simulink model "untitled1"  (R2022a)
settings: Solver=ode4  StartTime=0.0  StopTime=50000  FixedStep=1  RelTol=1e-3
libraries: nesl_utility x13, sm_lib x11, sharedtransform x4, sharedutil x1
settings Model: Creator=sakur  LastModifiedBy=sakur

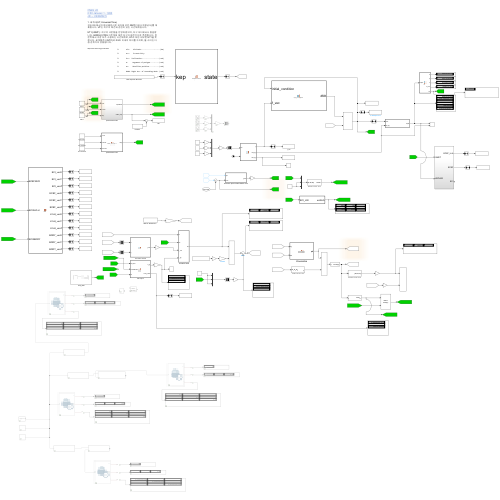
[thumbnail: Simulink's stored preview of the top-level diagram]
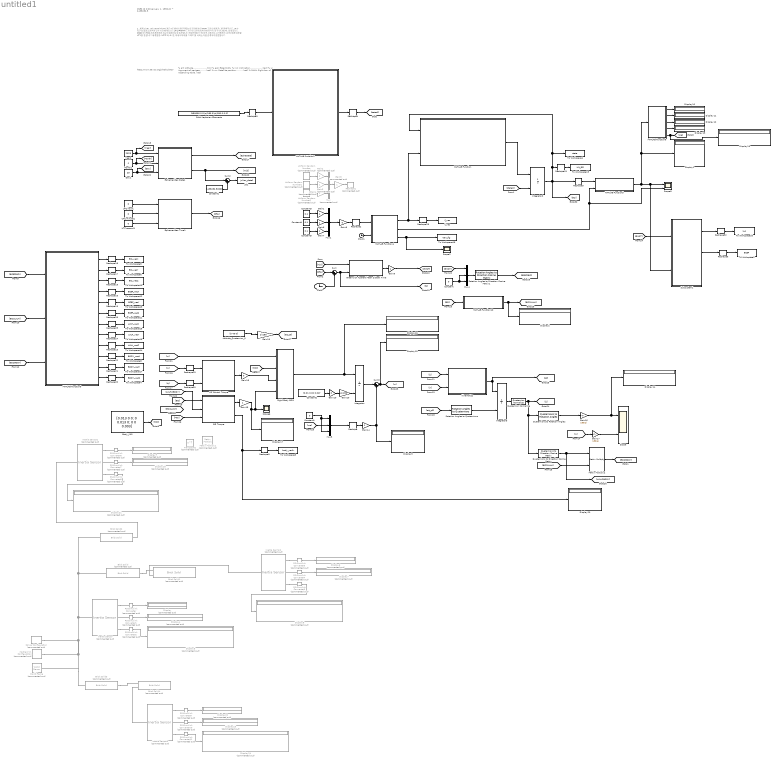
== system untitled1 ==
  note: % alt: Altitude.....................(Km)
      | % ecc: Eccentricity
      | % inc: Inclination...................(rad)
      | % w: Argument of perigee..........(rad)
      | % nu: Satellite position...........(rad) % RAAN: Right Asc. of Ascending Node. (rad)
  note: 1. 세계시(UT, Universal Time)
      | 경도 0도에서의 평균태양시로 과거에 쓰던 GMT(그리니치평균시)를 대체합니다. UT는 지구의 회전과 관련이 있는 시간체계입니다.
      |
      | UT1(=GMT) : 지구의 극운동을 반영하였으며, 지구 어디에서나 동일합니다. GCRS와 ITRS 기준계에 대한 지구의 회전각으로 측정합니다. 천문학에서 가장 자주 사용하는 시간체계로, UT라 하면 대부분 UT1을 뜻합니다. 세계협정시(UTC)와 0.9초 이내의 차이를 가지며, 둘 사이는 다음 관계식이 성립됩니다.
  note: CNES JD
      | 0:00 January 1, 1950
      | JD − 2433282.5
  note: https://www.aavso.org/jd-calculator
  Attitude_Quaternion_0 : Constant  Value=[0 45 0]'
  Body_MOI : Constant  Value=[0.013 0 0; 0 0.013 0; 0 0 0.003]
  Brick Solid : sm_lib/Body Elements/Brick Solid  Commented=on  GraphicAmbientColor=[0.15 0.15 0.15 1.0]  BasedOnType=Mass  BrickDimensions=[10 10 10]  BrickDimensionUnits=cm  CenterOfMass=[0 0 0]  CenterOfMassUnits=m  GraphicDiffuseColor=[0.5 0.5 0.5]  Density=1000  DensityUnits=kg/m^3  DoExposeReferenceFrame=on  GraphicEmissiveColor=[0.0 0.0 0.0 1.0]  ExportEntireGeometry=off  SerializedFrames=<Frames><Frame><Id>Frame1</Id><Value><Name>MS_Mount_F</Name><Origin><Source>GeometricFeature</Source><FeatureName>+z surface</FeatureName></Origin><PrimaryAxis><DefinedDirection>+Z</DefinedDirection><Source>ReferenceFrame</Source><SourceDirection>+Z</SourceDirection><FeatureName></FeatureName></PrimaryAxis><SecondaryAxis><DefinedDirection>+X</DefinedDirection><Source>ReferenceFrame</Source><SourceDirection>+X</SourceDirection><FeatureName></FeatureName></SecondaryAxis></Value></Frame></Frames>  MarkerShape=Sphere  MarkerSize=10  GraphicType=FromGeometry  InertiaType=CalculateFromGeometry  Mass=10  MassUnits=kg  MomentsOfInertia=[1 1 1]  MomentsOfInertiaUnits=kg*m^2  GraphicOpacity=1.0  ProductsOfInertia=[0 0 0]  ProductsOfInertiaUnits=kg*m^2  GraphicShininess=75  GraphicSpecularColor=[0.5 0.5 0.5 1.0]  GraphicVisPropType=SimpleVisualProperties
  Brick Solid1 : sm_lib/Body Elements/Brick Solid  Commented=on  GraphicAmbientColor=[0.15 0.15 0.15 1.0]  BasedOnType=Mass  BrickDimensions=[10 10 20]  BrickDimensionUnits=cm  CenterOfMass=[0 0 0]  CenterOfMassUnits=m  GraphicDiffuseColor=[0.5 0.5 0.5]  Density=1000  DensityUnits=kg/m^3  DoExposeReferenceFrame=on  GraphicEmissiveColor=[0.0 0.0 0.0 1.0]  ExportEntireGeometry=off  SerializedFrames=<Frames><Frame><Id>Frame1</Id><Value><Name>Mount_F</Name><Origin><Source>GeometricFeature</Source><FeatureName>-z surface</FeatureName></Origin><PrimaryAxis><DefinedDirection>+Z</DefinedDirection><Source>ReferenceFrame</Source><SourceDirection>+Z</SourceDirection><FeatureName></FeatureName></PrimaryAxis><SecondaryAxis><DefinedDirection>+X</DefinedDirection><Source>ReferenceFrame</Source><SourceDirection>+X</SourceDirection><FeatureName></FeatureName></SecondaryAxis></Value></Frame><Frame><Id>Frame2</Id><Value><Name>MOI_F</Name><Origin><Source>CenterOfMassFrame</Source><FeatureName></FeatureName></Origin><PrimaryAxis><DefinedDirection>-Z</DefinedDirection><Source>ReferenceFrame</Source><SourceDirection>+Z</SourceDirection><FeatureName></FeatureName></PrimaryAxis><SecondaryAxis><DefinedDirection>+X</DefinedDirection><Source>ReferenceFrame</Source><SourceDirection>+X</SourceDirection><FeatureName></FeatureName></SecondaryAxis></Value></Frame></Frames>  MarkerShape=Sphere  MarkerSize=10  GraphicType=FromGeometry  InertiaType=CalculateFromGeometry  Mass=2  MassUnits=kg  MomentsOfInertia=[1 1 1]  MomentsOfInertiaUnits=kg*m^2  GraphicOpacity=1.0  ProductsOfInertia=[0 0 0]  ProductsOfInertiaUnits=kg*m^2  GraphicShininess=75  GraphicSpecularColor=[0.5 0.5 0.5 1.0]  GraphicVisPropType=SimpleVisualProperties
  Brick Solid2 : sm_lib/Body Elements/Brick Solid  Commented=on  GraphicAmbientColor=[0.15 0.15 0.15 1.0]  BasedOnType=Mass  BrickDimensions=[10 10 30]  BrickDimensionUnits=cm  CenterOfMass=[0 0 0]  CenterOfMassUnits=m  GraphicDiffuseColor=[0.5 0.5 0.5]  Density=1000  DensityUnits=kg/m^3  DoExposeReferenceFrame=on  GraphicEmissiveColor=[0.0 0.0 0.0 1.0]  ExportEntireGeometry=off  SerializedFrames=<Frames><Frame><Id>Frame1</Id><Value><Name>MS_Mount_F</Name><Origin><Source>GeometricFeature</Source><FeatureName>+z surface</FeatureName></Origin><PrimaryAxis><DefinedDirection>+Z</DefinedDirection><Source>ReferenceFrame</Source><SourceDirection>+Z</SourceDirection><FeatureName></FeatureName></PrimaryAxis><SecondaryAxis><DefinedDirection>+X</DefinedDirection><Source>ReferenceFrame</Source><SourceDirection>+X</SourceDirection><FeatureName></FeatureName></SecondaryAxis></Value></Frame></Frames>  MarkerShape=Sphere  MarkerSize=10  GraphicType=FromGeometry  InertiaType=CalculateFromGeometry  Mass=12  MassUnits=kg  MomentsOfInertia=[1 1 1]  MomentsOfInertiaUnits=kg*m^2  GraphicOpacity=1.0  ProductsOfInertia=[0 0 0]  ProductsOfInertiaUnits=kg*m^2  GraphicShininess=75  GraphicSpecularColor=[0.5 0.5 0.5 1.0]  GraphicVisPropType=SimpleVisualProperties
  Brick Solid3 : sm_lib/Body Elements/Brick Solid  Commented=on  GraphicAmbientColor=[0.15 0.15 0.15 1.0]  BasedOnType=Mass  BrickDimensions=[10 10 10]  BrickDimensionUnits=cm  CenterOfMass=[0 0 0]  CenterOfMassUnits=m  GraphicDiffuseColor=[0.5 0.5 0.5]  Density=1000  DensityUnits=kg/m^3  DoExposeReferenceFrame=on  GraphicEmissiveColor=[0.0 0.0 0.0 1.0]  ExportEntireGeometry=off  SerializedFrames=<Frames><Frame><Id>Frame1</Id><Value><Name>MS_Mount_F</Name><Origin><Source>GeometricFeature</Source><FeatureName>+z surface</FeatureName></Origin><PrimaryAxis><DefinedDirection>+Z</DefinedDirection><Source>ReferenceFrame</Source><SourceDirection>+Z</SourceDirection><FeatureName></FeatureName></PrimaryAxis><SecondaryAxis><DefinedDirection>+X</DefinedDirection><Source>ReferenceFrame</Source><SourceDirection>+X</SourceDirection><FeatureName></FeatureName></SecondaryAxis></Value></Frame></Frames>  MarkerShape=Sphere  MarkerSize=10  GraphicType=FromGeometry  InertiaType=CalculateFromGeometry  Mass=10  MassUnits=kg  MomentsOfInertia=[1 1 1]  MomentsOfInertiaUnits=kg*m^2  GraphicOpacity=1.0  ProductsOfInertia=[0 0 0]  ProductsOfInertiaUnits=kg*m^2  GraphicShininess=75  GraphicSpecularColor=[0.5 0.5 0.5 1.0]  GraphicVisPropType=SimpleVisualProperties
  Brick Solid4 : sm_lib/Body Elements/Brick Solid  Commented=on  GraphicAmbientColor=[0.15 0.15 0.15 1.0]  BasedOnType=Mass  BrickDimensions=[10 10 10]  BrickDimensionUnits=cm  CenterOfMass=[0 0 0]  CenterOfMassUnits=m  GraphicDiffuseColor=[0.5 0.5 0.5]  Density=1000  DensityUnits=kg/m^3  DoExposeReferenceFrame=on  GraphicEmissiveColor=[0.0 0.0 0.0 1.0]  ExportEntireGeometry=off  SerializedFrames=<Frames><Frame><Id>Frame1</Id><Value><Name>MS_Mount_F</Name><Origin><Source>GeometricFeature</Source><FeatureName>-z surface</FeatureName></Origin><PrimaryAxis><DefinedDirection>+Z</DefinedDirection><Source>ReferenceFrame</Source><SourceDirection>+Z</SourceDirection><FeatureName></FeatureName></PrimaryAxis><SecondaryAxis><DefinedDirection>+X</DefinedDirection><Source>ReferenceFrame</Source><SourceDirection>+X</SourceDirection><FeatureName></FeatureName></SecondaryAxis></Value></Frame><Frame><Id>Frame2</Id><Value><Name>MoI_F</Name><Origin><Source>CenterOfMassFrame</Source><FeatureName></FeatureName></Origin><PrimaryAxis><DefinedDirection>-Z</DefinedDirection><Source>ReferenceFrame</Source><SourceDirection>+Z</SourceDirection><FeatureName></FeatureName></PrimaryAxis><SecondaryAxis><DefinedDirection>+X</DefinedDirection><Source>ReferenceFrame</Source><SourceDirection>+X</SourceDirection><FeatureName></FeatureName></SecondaryAxis></Value></Frame></Frames>  MarkerShape=Sphere  MarkerSize=10  GraphicType=FromGeometry  InertiaType=CalculateFromGeometry  Mass=10  MassUnits=kg  MomentsOfInertia=[1 1 1]  MomentsOfInertiaUnits=kg*m^2  GraphicOpacity=1.0  ProductsOfInertia=[0 0 0]  ProductsOfInertiaUnits=kg*m^2  GraphicShininess=75  GraphicSpecularColor=[0.5 0.5 0.5 1.0]  GraphicVisPropType=SimpleVisualProperties
  Clock : Clock
  Clock1 : Clock
  Constant : Constant  Value=0
  Constant1 : Constant  Value=0
  Constant2 : Constant  Value=[0.01 0.02 0.01]'
  Constant3 : Constant  Value=0.1
  Constant4 : Constant  Value=0.1
  Constant5 : Constant  Value=0.1
  Day1 : Constant  Value=25
  Display{,4..9,18,21..24} (12 alike) : Display  Commented=on
  Display{1..3,10..17,19..20} (13 alike) : Display
  Ephemerides Date1 : Subsystem
  Ephemerides Time1 : MATLAB Function  TreatAsAtomicUnit=on
  GG Torque : MATLAB Function  TreatAsAtomicUnit=on
  Gain{1,6..7,9,14..15} (6 alike) : Gain
  Gain10 : Gain  Gain=0
  Gain16 : Gain  Gain=180/pi
  Gain17 : Gain  Gain=180/pi
  Gain18 : Gain  Gain=0
  Gain19 : Gain  Gain=pi/180
  Gain{2..5} (4 alike) : Gain  Commented=on
  Gain20 : Gain  Gain=pi/180
  Gain8 : Gain  Gain=0
  Greenwich Aparent Mean Sideral Time : MATLAB Function  TreatAsAtomicUnit=on
  Inertia Sensor : sm_lib/Body Elements/Inertia Sensor  Commented=on  SensorExtent=Mechanism  SpanWeldJoints=off  ExcludeGroundedBodies=off  MeasurementFrame=World  SenseMass=on  SenseCenterOfMass=on  SenseInertiaMatrix=on  SenseCenteredInertiaMatrix=off  SensePrincipalInertiaMatrix=off  SenseRotationMatrix=off  GraphicType=PrincipalInertiaFrame  PrincipalInertiaFrameSize=20  GraphicVisPropType=SimpleVisualProperties  GraphicDiffuseColor=[0.5 0.5 0.5]  GraphicSpecularColor=[0.5 0.5 0.5 1.0]  GraphicAmbientColor=[0.15 0.15 0.15 1.0]  GraphicEmissiveColor=[0.0 0.0 0.0 1.0]  GraphicShininess=75  GraphicOpacity=1.0
      settings: SourceProductBaseCode=MS
  Inertia Sensor1 : sm_lib/Body Elements/Inertia Sensor  Commented=on  SensorExtent=Mechanism  SpanWeldJoints=off  ExcludeGroundedBodies=off  MeasurementFrame=Attached  SenseMass=on  SenseCenterOfMass=on  SenseInertiaMatrix=on  SenseCenteredInertiaMatrix=off  SensePrincipalInertiaMatrix=off  SenseRotationMatrix=off  GraphicType=PrincipalInertiaFrame  PrincipalInertiaFrameSize=20  GraphicVisPropType=SimpleVisualProperties  GraphicDiffuseColor=[0.5 0.5 0.5]  GraphicSpecularColor=[0.5 0.5 0.5 1.0]  GraphicAmbientColor=[0.15 0.15 0.15 1.0]  GraphicEmissiveColor=[0.0 0.0 0.0 1.0]  GraphicShininess=75  GraphicOpacity=1.0
      settings: SourceProductBaseCode=MS
  Inertia Sensor2 : sm_lib/Body Elements/Inertia Sensor  Commented=on  SensorExtent=Mechanism  SpanWeldJoints=off  ExcludeGroundedBodies=off  MeasurementFrame=World  SenseMass=on  SenseCenterOfMass=on  SenseInertiaMatrix=on  SenseCenteredInertiaMatrix=off  SensePrincipalInertiaMatrix=off  SenseRotationMatrix=off  GraphicType=PrincipalInertiaFrame  PrincipalInertiaFrameSize=20  GraphicVisPropType=SimpleVisualProperties  GraphicDiffuseColor=[0.5 0.5 0.5]  GraphicSpecularColor=[0.5 0.5 0.5 1.0]  GraphicAmbientColor=[0.15 0.15 0.15 1.0]  GraphicEmissiveColor=[0.0 0.0 0.0 1.0]  GraphicShininess=75  GraphicOpacity=1.0
      settings: SourceProductBaseCode=MS
  Inertia Sensor3 : sm_lib/Body Elements/Inertia Sensor  Commented=on  SensorExtent=Mechanism  SpanWeldJoints=off  ExcludeGroundedBodies=off  MeasurementFrame=Attached  SenseMass=on  SenseCenterOfMass=on  SenseInertiaMatrix=on  SenseCenteredInertiaMatrix=off  SensePrincipalInertiaMatrix=off  SenseRotationMatrix=off  GraphicType=PrincipalInertiaFrame  PrincipalInertiaFrameSize=20  GraphicVisPropType=SimpleVisualProperties  GraphicDiffuseColor=[0.5 0.5 0.5]  GraphicSpecularColor=[0.5 0.5 0.5 1.0]  GraphicAmbientColor=[0.15 0.15 0.15 1.0]  GraphicEmissiveColor=[0.0 0.0 0.0 1.0]  GraphicShininess=75  GraphicOpacity=1.0
      settings: SourceProductBaseCode=MS
  Integrator : Integrator  InitialConditionSource=external
  Integrator2 : Integrator  InitialConditionSource=external  InitialCondition=[-7000 0 0 0 -9.175045 0 5233.5]'
  Integrator3 : Integrator  InitialConditionSource=external
  JD1 : ToWorkspace  VariableName=Julian_date1  SampleTime=-1
  Kinematics : MATLAB Function  TreatAsAtomicUnit=on
  MATLAB Function : MATLAB Function  TreatAsAtomicUnit=on
  MATLAB Function10 : MATLAB Function  TreatAsAtomicUnit=on
  MATLAB Function2 : MATLAB Function  TreatAsAtomicUnit=on
  MATLAB Function4 : MATLAB Function  TreatAsAtomicUnit=on
  MATLAB Function5 : MATLAB Function  TreatAsAtomicUnit=on
  MATLAB Function8 : MATLAB Function  TreatAsAtomicUnit=on
  MATLAB Function9 : MATLAB Function  TreatAsAtomicUnit=on
  Matrix Multiply1 : Product  Commented=on  Multiplication=Matrix(*)
  Matrix Multiply2 : Product  Multiplication=Matrix(*)
  Mechanism Configuration : sm_lib/Utilities/Mechanism Configuration  Commented=on  UniformGravity=None  GravityVector=[0 0 -9.80665]  GravityUnits=m/s^2  LinearizationDelta=0.001  JointModeTransitionNonlinearIterations=2
  Month1 : Constant  Value=4
  Mux : Mux  Commented=on  Inputs=3
  Mux1 : Mux  Inputs=3
  Mux4 : Mux  Inputs=3
  Mux5 : Mux  Inputs=3
  Orbit Keplerian Elements : Constant  Value=[450000 0 0*pi/180 0*pi/180 0 0 0]
  PD Control Torque : MATLAB Function  TreatAsAtomicUnit=on
  PS-Simulink Converter{,1..11} (12 alike) : nesl_utility/PS-Simulink Converter  Commented=on  PhysicalDomain=network_engine_domain  SubClassName=ps_output  LeftPortType=input  RightPortType=output  PseudoPeriodic=off  Frequencies=[]  VectorFormat=inherit  Unit=inherit  AffineConversion=off
      settings: SourceProductBaseCode=SS,PW,VE
  Quaternion Normalize : sharedutil/Quaternion Normalize  aMode=aMode
      settings: SourceProductBaseCode=AE,PW,DR,MT,VE
  Quaternions to Direction Cosine Matrix : sharedtransform/Quaternions to  Direction Cosine Matrix  aMode=aMode
      settings: SourceProductBaseCode=AE,PW,DR,MT,VE
  Quaternions to Rotation Angles : sharedtransform/Quaternions to Rotation Angles  rotationOrder=ZYX  aMode=aMode
      settings: SourceProductBaseCode=AE,PW,DR,MT,VE
  Reshape{,2,29..30} (4 alike) : Reshape  OutputDimensionality=Column vector (2-D)
  Reshape1 : Reshape  Commented=on  OutputDimensionality=Column vector (2-D)
  Reshape{3..6,9,13,16..26,28,31..32} (20 alike) : Reshape  OutputDimensionality=Row vector (2-D)
  Rigid Body EOM : MATLAB Function  TreatAsAtomicUnit=on
  Rotation Angles to Direction Cosine Matrix1 : sharedtransform/Rotation Angles to Direction Cosine Matrix  rotationOrder=ZYX  aMode=aMode
      settings: SourceProductBaseCode=AE,PW,DR,MT,VE
  Rotation Angles to Quaternions : sharedtransform/Rotation Angles to Quaternions  rotationOrder=ZYX  aMode=aMode
      settings: SourceProductBaseCode=AE,PW,DR,MT,VE
  Scope : Scope  NumInputPorts=2
  Scope2 : Scope
  Scope5 : Scope  NumInputPorts=2
  Scope6 : Scope
  Solver Configuration : nesl_utility/Solver Configuration  Commented=on  PhysicalDomain=network_engine_domain  SubClassName=solver  LeftPortType=input  RightPortType=generic  Tones=[]  Harmonics=[]  SimulateNoise=off  Profile=off  UseLocalSampling=off  EnableSwitchedLinearOptims=on  FrequencyDomain=off  UseCCode=off  RelTol=0.001  AbsTol=0.001  MinStep=1e-09  ToWorkspace=off  RevertToSquareIcSolve=off  NumHomotopyIterations=100  PhasorMode=off  PhasorModeNumHarmonics=1  IndexReductionMethod=DerivativeReplacement  DoDC=off  ResidualTolerance=1e-09  UseLocalSolver=off  LocalSolverChoice=NE_BACKWARD_EULER_ADVANCER  LocalSolverSampleTime=0.001  DoFixedCost=off  MaxNonlinIter=3  MaxModeIter=2  ComputeImpulses=off  ImpulseIterations=2  LinearAlgebra=auto  LinearAlgebraNumThread=0  EquationFormulation=NE_TIME_EF  DelaysMemoryBudget=1024  AutomaticFiltering=on  FilteringTimeConstant=0.001  PartitionStorageMethod=AS_NEEDED  PartitionMemoryBudget=1024  PartitionMethod=ROBUST
      settings: SourceProductBaseCode=SS,PW,VE
  Subsystem1 : Subsystem
  Sum : Sum  Inputs=|++
  Sum2 : Sum  Inputs=|++
  Sum3 : Sum  Inputs=|++
  To Workspace1 : ToWorkspace  VariableName=state  SampleTime=-1
      settings: Save2DSignal=2-D array (concatenate along first dimension)
  To Workspace10 : ToWorkspace  VariableName=ECI_vecZ  SampleTime=-1
      settings: Save2DSignal=2-D array (concatenate along first dimension)
  To Workspace11 : ToWorkspace  VariableName=ECEF_vecZ  SampleTime=-1
      settings: Save2DSignal=2-D array (concatenate along first dimension)
  To Workspace12 : ToWorkspace  VariableName=ECEF_vecX  SampleTime=-1
      settings: Save2DSignal=2-D array (concatenate along first dimension)
  To Workspace13 : ToWorkspace  VariableName=ECEF_vecY  SampleTime=-1
      settings: Save2DSignal=2-D array (concatenate along first dimension)
  To Workspace14 : ToWorkspace  VariableName=LVLH_vecZ  SampleTime=-1
      settings: Save2DSignal=2-D array (concatenate along first dimension)
  To Workspace15 : ToWorkspace  VariableName=LVLH_vecX  SampleTime=-1
      settings: Save2DSignal=2-D array (concatenate along first dimension)
  To Workspace16 : ToWorkspace  VariableName=LVLH_vecY  SampleTime=-1
      settings: Save2DSignal=2-D array (concatenate along first dimension)
  To Workspace17 : ToWorkspace  VariableName=BODY_vecY  SampleTime=-1
      settings: Save2DSignal=2-D array (concatenate along first dimension)
  To Workspace18 : ToWorkspace  VariableName=tran_flg  SampleTime=-1
      settings: Save2DSignal=2-D array (concatenate along first dimension)
  To Workspace19 : ToWorkspace  VariableName=LIN_ECI  SampleTime=-1
      settings: Save2DSignal=2-D array (concatenate along first dimension)
  To Workspace2 : ToWorkspace  VariableName=ECEF  SampleTime=-1
      settings: Save2DSignal=2-D array (concatenate along first dimension)
  To Workspace20 : ToWorkspace  VariableName=LLA  SampleTime=-1
      settings: Save2DSignal=2-D array (concatenate along first dimension)
  To Workspace4 : ToWorkspace  VariableName=BODY_vecZ  SampleTime=-1
      settings: Save2DSignal=2-D array (concatenate along first dimension)
  To Workspace5 : ToWorkspace  VariableName=ECI_vecX  SampleTime=-1
      settings: Save2DSignal=2-D array (concatenate along first dimension)
  To Workspace6 : ToWorkspace  VariableName=ECI_vecY  SampleTime=-1
      settings: Save2DSignal=2-D array (concatenate along first dimension)
  To Workspace8 : ToWorkspace  VariableName=BODY_vecX  SampleTime=-1
      settings: Save2DSignal=2-D array (concatenate along first dimension)
  To Workspace9 : ToWorkspace  VariableName=body_nadir  SampleTime=-1
      settings: Save2DSignal=2-D array (concatenate along first dimension)
  Transpose2 : Math  Commented=on  Operator=transpose
  UTC hour1 : Constant  Value=0
  UTC minute1 : Constant  Value=0
  UTC second1 : Constant  Value=0
  Uniform Random Number : UniformRandomNumber  Commented=on  Minimum=-0.5  Maximum=0.5  SampleTime=1
  Uniform Random Number1 : UniformRandomNumber  Commented=on  Minimum=-0.5  Maximum=0.5  SampleTime=1
  Uniform Random Number2 : UniformRandomNumber  Commented=on  Minimum=-0.5  Maximum=0.5  SampleTime=1
  World Frame : sm_lib/Frames and Transforms/World Frame  Commented=on
  Year1 : Constant  Value=2023
  constant1 : Constant  Value=2433282.50000
  f_vec : ToWorkspace  VariableName=f_vec  SampleTime=-1
      settings: Save2DSignal=2-D array (concatenate along first dimension)
  wires:
  MATLAB Function2/1(state) -> Reshape4/1
  Reshape3/1 -> MATLAB Function2/1(kep)
  Reshape4/1 -> [state0]
  [state0] -> Integrator2/2
  MATLAB Function/1(dfdt) -> Integrator2/1
  MATLAB Function5/1(kepel) -> MATLAB Function8/1(kepler), Display1/1, Subsystem1/2(KEPLER), Scope5/1
  Reshape5/1 -> MATLAB Function5/1(statv)
  Uniform Random Number/1 -> Gain2/1
  Uniform Random Number1/1 -> Gain3/1
  Uniform Random Number2/1 -> Gain4/1
  Gain2/1 -> Mux/1
  Gain3/1 -> Mux/2
  Gain4/1 -> Mux/3
  Mux/1 -> Gain5/1
  MATLAB Function4/1(y) -> MATLAB Function/2(f_vec), Reshape28/1
  Gain5/1 -> Reshape1/1
  MATLAB Function4/2(kep_flg) -> Scope5/2, MATLAB Function5/2(kep_flg)
  Clock1/1 -> MATLAB Function4/2(t)
  Mux1/1 -> Gain8/1
  Constant4/1 -> Gain6/1
  Gain8/1 -> Reshape2/1
  Gain7/1 -> Mux1/3
  Gain1/1 -> Mux1/1
  Gain6/1 -> Mux1/2
  Constant5/1 -> Gain7/1
  Constant3/1 -> Gain1/1
  Reshape2/1 -> MATLAB Function4/1(vec)
  Clock/1 -> Sum/2
  Sum/1 -> Greenwich Aparent Mean Sideral Time/2(time), [ts]
  Greenwich Aparent Mean Sideral Time/1(gwst) -> Gain9/1
  [mjd] -> Greenwich Aparent Mean Sideral Time/1(diju)
  [dfra] -> Sum/1
  Gain9/1 -> [GMST]
  Reshape23/1 -> To Workspace14/1
  MATLAB Function9/5(ECEF_vecY) -> Reshape13/1
  Reshape26/1 -> To Workspace11/1
  [ECI2BODY] -> MATLAB Function9/3(ECI2BODY)
  Reshape18/1 -> To Workspace5/1
  MATLAB Function9/10(BODY_vecX) -> Reshape22/1
  MATLAB Function9/9(LVLH_vecZ) -> Reshape23/1
  Reshape25/1 -> To Workspace15/1
  MATLAB Function9/1(ECI_vecX) -> Reshape18/1
  [ECEF2ECI] -> MATLAB Function9/1(ECEF2ECI)
  Reshape24/1 -> To Workspace16/1
  MATLAB Function9/3(ECI_vecZ) -> Reshape19/1
  [ECI2LVLH] -> MATLAB Function9/2(ECI2LVLH)
  MATLAB Function9/6(ECEF_vecZ) -> Reshape26/1
  MATLAB Function9/11(BODY_vecY) -> Reshape21/1
  Reshape21/1 -> To Workspace17/1
  Reshape20/1 -> To Workspace4/1
  MATLAB Function9/2(ECI_vecY) -> Reshape17/1
  MATLAB Function9/12(BODY_vecZ) -> Reshape20/1
  MATLAB Function9/4(ECEF_vecX) -> Reshape16/1
  Reshape17/1 -> To Workspace6/1
  MATLAB Function9/8(LVLH_vecY) -> Reshape24/1
  Reshape22/1 -> To Workspace8/1
  Reshape16/1 -> To Workspace12/1
  Reshape19/1 -> To Workspace10/1
  MATLAB Function9/7(LVLH_vecX) -> Reshape25/1
  Reshape13/1 -> To Workspace13/1
  Sum2/1 -> JD1/1
  constant1/1 -> Sum2/2
  Ephemerides Date1/1(EpheDate) -> [EpheDate]
  Month1/1 -> [Month], Ephemerides Date1/2(month)  "month"
  Ephemerides Date1/2(CNES_mdj) -> Sum2/1, [mjd]
  UTC minute1/1 -> Ephemerides Time1/2(minutes)
  Ephemerides Time1/1(dayf) -> [dfra]
  Year1/1 -> Ephemerides Date1/1(year), [Year]  "year"
  UTC second1/1 -> Ephemerides Time1/3(seconds)
  Day1/1 -> [Day], Ephemerides Date1/3(day)  "date"
  UTC hour1/1 -> Ephemerides Time1/1(hours)
  Orbit Keplerian Elements/1 -> Reshape3/1
  MATLAB Function4/3(tran_flg) -> Scope2/1, To Workspace18/1
  Reshape28/1 -> f_vec/1
  MATLAB Function8/1(ra) -> Display10/1
  MATLAB Function8/2(rp) -> Display11/1
  MATLAB Function8/3(T) -> Display12/1
  MATLAB Function8/4(T_hour) -> Display13/1
  Mux5/1 -> Reshape/1
  [q] -> Kinematics/1(q)
  [q] -> Reshape30/1
  Gain15/1 -> Rigid Body EOM/4(t_gg), Scope6/1, Display17/1
  [att_q0] -> Rotation Angles to Quaternions/1
  Rotation Angles to Quaternions/1 -> Integrator3/2
  [w] -> Reshape29/1
  [w] -> Rigid Body EOM/1(w)
  Gain17/1 -> Scope/2
  Quaternions to Rotation Angles/1 -> Gain16/1
  [ECI] -> GG Torque/1(LIN_ECI)
  GG Torque/1(t_gg) -> Gain15/1
  [w] -> Gain17/1
  Reshape30/1 -> PD Control Torque/2(q)
  PD Control Torque/1(t_cntl) -> Gain18/1
  Reshape29/1 -> PD Control Torque/1(w)
  Gain18/1 -> Rigid Body EOM/3(t_cntl)
  Gain16/1 -> Display14/1, Scope/1
  Integrator3/1 -> Quaternion Normalize/1
  Integrator/1 -> Sum3/1
  Quaternion Normalize/1 -> Quaternions to Direction Cosine Matrix/1, Quaternions to Rotation Angles/1, [q]
  Sum3/1 -> Display15/1, [w]
  [w] -> Kinematics/2(w)
  Gain14/1 -> Display3/1, Sum3/2
  Constant2/1 -> Gain10/1
  Rigid Body EOM/1(wd) -> Integrator/1, Display16/1
  Kinematics/1(qd) -> Integrator3/1, [qd]
  Attitude_Quaternion_0/1 -> Gain19/1
  Constant/1 -> Mux4/2, Mux4/3
  [GMST] -> Mux4/1
  Mux4/1 -> Rotation Angles to Direction Cosine Matrix1/1
  Rotation Angles to Direction Cosine Matrix1/1 -> [ECEF2ECI]
  MATLAB Function10/1(eci2lvlh) -> Display2/1, [ECI2LVLH]
  [ECI] -> MATLAB Function10/1(ECI_LIN)
  Integrator2/1 -> [ECI], To Workspace1/1, MATLAB Function/1(initial_condition), Reshape31/1, Reshape5/1
  Reshape31/1 -> To Workspace19/1
  [GMST] -> Subsystem1/1(GMST)
  Reshape32/1 -> To Workspace20/1
  Subsystem1/1(ECEF_LLA) -> Reshape32/1
  Reshape6/1 -> To Workspace2/1
  Subsystem1/2(ECEF) -> Reshape6/1
  MATLAB Function8/5(we) -> Display19/1, [we]
  Constant1/1 -> Mux5/1, Mux5/3
  [we] -> Mux5/2
  Reshape/1 -> Gain14/1
  Gain19/1 -> [att_q0]
  Body_MOI/1 -> [MOI]
  [MOI] -> GG Torque/3(Jb)
  [MOI] -> Rigid Body EOM/2(Jb)
  Reshape9/1 -> To Workspace9/1
  GG Torque/2(body_nadir) -> Display20/1, Reshape9/1
  [LVLH2BODY] -> GG Torque/2(LVLH2BODY)
  Quaternions to Direction Cosine Matrix/1 -> [LVLH2BODY], Matrix Multiply2/1
  Matrix Multiply2/1 -> [ECI2BODY]
  [ECI2LVLH] -> Matrix Multiply2/2
  Gain20/1 -> Integrator/2
  Gain10/1 -> Gain20/1
  PS-Simulink Converter/1 -> Display/1
  PS-Simulink Converter1/1 -> Display4/1
  PS-Simulink Converter2/1 -> Display5/1
  PS-Simulink Converter5/1 -> Display8/1
  PS-Simulink Converter4/1 -> Display7/1
  PS-Simulink Converter3/1 -> Display6/1
  PS-Simulink Converter7/1 -> Display18/1
  PS-Simulink Converter6/1 -> Display9/1
  PS-Simulink Converter8/1 -> Display21/1
  PS-Simulink Converter11/1 -> Display24/1
  PS-Simulink Converter10/1 -> Display23/1
  PS-Simulink Converter9/1 -> Display22/1
  connections:
  Inertia Sensor/RConn1 -- PS-Simulink Converter/LConn1
  PS-Simulink Converter1/LConn1 -- Inertia Sensor/RConn2
  Inertia Sensor/RConn3 -- PS-Simulink Converter2/LConn1
  Inertia Sensor1/RConn3 -- PS-Simulink Converter5/LConn1
  PS-Simulink Converter4/LConn1 -- Inertia Sensor1/RConn2
  Inertia Sensor1/RConn1 -- PS-Simulink Converter3/LConn1
  Inertia Sensor2/RConn3 -- PS-Simulink Converter8/LConn1
  PS-Simulink Converter7/LConn1 -- Inertia Sensor2/RConn2
  Inertia Sensor2/RConn1 -- PS-Simulink Converter6/LConn1
  Inertia Sensor2/LConn1 -- Brick Solid2/LConn1
  Brick Solid/LConn1 -- Brick Solid1/LConn1
  Brick Solid1/LConn2 -- Inertia Sensor1/LConn1
  Solver Configuration/RConn1 -- Brick Solid3/RConn1 -- World Frame/RConn1 -- Mechanism Configuration/RConn1 -- Brick Solid/RConn1 -- Brick Solid2/RConn1 -- Inertia Sensor/LConn1
  Inertia Sensor3/RConn3 -- PS-Simulink Converter11/LConn1
  PS-Simulink Converter10/LConn1 -- Inertia Sensor3/RConn2
  Inertia Sensor3/RConn1 -- PS-Simulink Converter9/LConn1
  Brick Solid3/LConn1 -- Brick Solid4/LConn1
  Brick Solid4/LConn2 -- Inertia Sensor3/LConn1

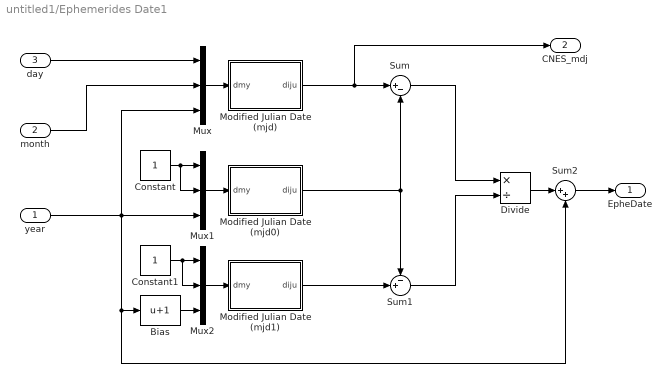
== system untitled1/Ephemerides Date1 ==
  year : Inport
  month : Inport  Port=2
  day : Inport  Port=3
  Bias : Bias  Bias=1  SaturateOnIntegerOverflow=off
  Constant : Constant
  Constant1 : Constant
  Divide : Product  Inputs=*/
  Modified Julian Date (mjd) : MATLAB Function  TreatAsAtomicUnit=on
  Modified Julian Date (mjd0) : MATLAB Function  TreatAsAtomicUnit=on
  Modified Julian Date (mjd1) : MATLAB Function  TreatAsAtomicUnit=on
  Mux : Mux  Inputs=3
  Mux1 : Mux  Inputs=3
  Mux2 : Mux  Inputs=3
  Sum : Sum  Inputs=|+-
  Sum1 : Sum  Inputs=-+|
  Sum2 : Sum  Inputs=|++
  EpheDate : Outport
  CNES_mdj : Outport  Port=2
  wires:
  Sum1/1 -> Divide/2
  Modified Julian Date (mjd1)/1(diju) -> Sum1/2
  month/1 -> Mux/2
  year/1 -> Mux1/3, Mux/3, Bias/1, Sum2/2
  Mux1/1 -> Modified Julian Date (mjd0)/1(dmy)
  day/1 -> Mux/1
  Mux/1 -> Modified Julian Date (mjd)/1(dmy)
  Mux2/1 -> Modified Julian Date (mjd1)/1(dmy)
  Bias/1 -> Mux2/3
  Modified Julian Date (mjd)/1(diju) -> CNES_mdj/1, Sum/1
  Constant1/1 -> Mux2/2, Mux2/1
  Sum/1 -> Divide/1
  Constant/1 -> Mux1/2, Mux1/1
  Modified Julian Date (mjd0)/1(diju) -> Sum1/1, Sum/2
  Divide/1 -> Sum2/1
  Sum2/1 -> EpheDate/1

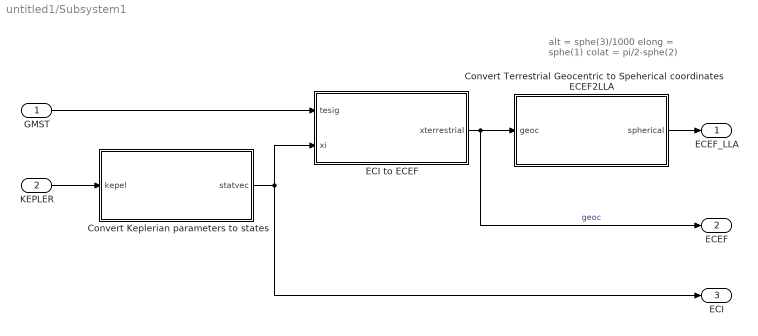
== system untitled1/Subsystem1 ==
  note: alt = sphe(3)/1000
      | elong = sphe(1)
      | colat = pi/2-sphe(2)
  GMST : Inport
  KEPLER : Inport  Port=2
  Convert Keplerian parameters to states : MATLAB Function  TreatAsAtomicUnit=on
  Convert Terrestrial Geocentric to Speherical coordinates ECEF2LLA : MATLAB Function  TreatAsAtomicUnit=on
  "ECI to ECEF " : MATLAB Function  TreatAsAtomicUnit=on
  ECEF_LLA : Outport
  ECEF : Outport  Port=2
  ECI : Outport  Port=3
  wires:
  "ECI to ECEF "/1(xterrestrial) -> ECEF/1, Convert Terrestrial Geocentric to Speherical coordinates ECEF2LLA/1(geoc)  "geoc"
  Convert Terrestrial Geocentric to Speherical coordinates ECEF2LLA/1(spherical) -> ECEF_LLA/1
  Convert Keplerian parameters to states/1(statvec) -> "ECI to ECEF "/2(xi), ECI/1
  GMST/1 -> "ECI to ECEF "/1(tesig)
  KEPLER/1 -> Convert Keplerian parameters to states/1(kepel)

== matlab function untitled1/Ephemerides Time1 ==
  data: hours input; dayf output; minutes input; seconds input
function dayf  = time_to_dayf(hours, minutes, seconds)
% [dayf] = time_to_dayf (hours, minutes, seconds)
%    The function time_to_dayf returns with the day elapesed
%    time in seconds
% inputs:
%   hours     
%       day hour (integer).
%   minutes
%       minutes (integer).
%   seconds
%       seconds and fraction of second
% outputs:
%   dayf
%       Day elapsed time in seconds. 
%
% Valdemir Carrara, Feb, 2009
%

dayf = seconds + 60*(minutes + 60*hours);

== matlab function untitled1/MATLAB Function8 ==
  data: kepler input; ra output; rp output; T output; T_hour output; we output
function [ra, rp, T, T_hour, we] = fcn(kepler)

u=3.9865*10^14;

a = kepler(1);
e = kepler(2);
% 

ra = a*(1+e);%장반경
rp = a*(1-e);%단반경

a = (ra+rp)/2;

% a = (550 + 6371.8)*1000;

T = 2*pi*sqrt((a*a*a)/(u));

T_hour = T/3600;

we = 2*pi/T;
% we = 1.1207*0.001;

end

== matlab function untitled1/GG Torque ==
  data: LIN_ECI input; t_gg output; LVLH2BODY input; Jb input; body_nadir output
function [t_gg, body_nadir] = fcn(LIN_ECI, LVLH2BODY, Jb)

r = LIN_ECI(1,1:3)';
r_ = r/norm(r);
R = norm(r);
mu = (3.986004418)*(10^14);

lvlh_nadir = [0 0 R]';

body_nadir = LVLH2BODY*lvlh_nadir;

% t_gg = 200000*(3*mu/(R^5))*cross(body_nadir, Jb*body_nadir);
t_gg = 200000*(3*mu/(R^5))*cross(body_nadir, Jb*body_nadir);


end

== matlab function untitled1/Kinematics ==
  data: q input; qd output; w input
function qd   = kinematics( q, w)
w1 = w(1);  w2 = w(2);  w3 = w(3);

Omega = [ 0 -w1 -w2 -w3; 
         w1   0  w3 -w2;
         w2 -w3   0  w1;
         w3  w2 -w1   0];

qd = 0.5*Omega*q;


end

== matlab function untitled1/PD Control Torque ==
  data: w input; t_cntl output; q input
function t_cntl = fcn(w, q)

K1 = diag([1 1 1]);
K2 = diag([1 1 1]);
q_ = q(2:4,1);

t_cntl = -K1*w + K2*q_;

end

== matlab function untitled1/Rigid Body EOM ==
  data: w input; Jb input; wd output; t_cntl input; t_gg input
function wd = fcn(w,Jb, t_cntl, t_gg)

t_dist = [0 0 0]';

% Jb = [10 0 0;
%       0 10 0;
%       0 0 10];

wd = inv(Jb)*(t_dist + t_cntl + t_gg - cross(w, Jb*w));

end

== matlab function untitled1/MATLAB Function10 ==
  data: ECI_LIN input; eci2lvlh output
function eci2lvlh  = fcn(ECI_LIN)
r = ECI_LIN(1:3)';
v = ECI_LIN(4:6)';

LVLH_Z = -r/norm(r);
LVLH_Y = -cross(v,LVLH_Z)/norm(cross(v,LVLH_Z));
LVLH_X =  cross(LVLH_Y, LVLH_Z);

eci2lvlh = [LVLH_X,LVLH_Y,LVLH_Z]';

end

== matlab function untitled1/Subsystem1/Convert Keplerian parameters to states ==
  data: kepel input; statvec output
function statvec = kepel_statvec(kepel)
%  [statvec] = kepel_statvec (kepel)
%	The function kepel_statvec transforms the keplerian
%	elements kepel into the corresponding state vector in
%	the same reference system.
%
% Input:
%	kepel
% 		vector containing the keplerian elements:
%		(1) - semimajor axis of the orbit in meters.
%		(2) - eccentricity.
%		(3) - inclination in radians.
%		(4) - right ascension of ascending node in radians.
%		(5) - argument of perigee in radians.
%		(6) - mean anomaly in radians.
%
% Output:
%	statvec
%  		state vector in meters and meters/second.
%
% Authors:
%	Helio K. Kuga;
%	Valder M. Medeiros;
%	Valdemir Carrara		february/80		version 1.0
%	Valdemir Carrara		july 2005		(C version)
%   Valdemir Carrara            March/09        Matlab

EARTH_GRAVITY	= 3.9860064e+14;		% Earth's gravitational constant (m**3/s**2)

a    = kepel(1);	% semi-major axis
exc  = kepel(2);	% eccentricity

c1   = sqrt(1. - exc*exc);

% Rotational matrix
rot_maz1 =  [cos(-kepel(4)), sin(-kepel(4)), 0;
             -sin(-kepel(4)), cos(-kepel(4)), 0; 
             0, 0, 1];
         
rot_max =  [1, 0, 0; 
           0, cos(-kepel(3)), sin(-kepel(3));
           0, -sin(-kepel(3)), cos(-kepel(3))];
       
rot_maz2 =  [cos(-kepel(5)), sin(-kepel(5)), 0;
             -sin(-kepel(5)), cos(-kepel(5)), 0; 
             0, 0, 1];
         
orb2iner = rot_maz1*rot_max*rot_maz2;

%%%%%%%%%%%%%%%%%%%%%%%%%%%%%%%%%%%%%%%%%%%%
%     Kepler's equation
%E    = kepler(kepel(6), exc);
mean_anomaly = kepel(6);
eccentricity = exc;
%function [eccentric] = kepler (mean_anomaly, eccentricity)
% [eccentric] = kepler (mean_anomaly, eccentricity)
%	The subroutine kepler finds a solution to the
%	kepler's equation.
%
% Input:
%	mean_anomaly
%		mean anomaly in radians.
%	eccentricity
%		eccentricity.
%
% Output:
%	eccentric
%		eccentric anomaly in radians.
%
% Authors:
%	Valder M. de Medeiros		june/81		version 2.0
%	Valdemir Carrara			july 2005	(C version)
%   Valdemir Carrara            March/09        Matlab

exc2    = eccentricity*eccentricity;
am1     = mod (mean_anomaly, 2*pi);
am2     = am1 + am1;
am3     = am1 + am2;
shoot   = am1 + eccentricity*(1. - 0.125*exc2)*sin(am1) + ...
		0.5*exc2*(sin(am2) + 0.75*eccentricity*sin(am3));
shoot   = mod (shoot, 2*pi);

e1      = 1.0;
ic      = 0;

while ((abs(e1) > 1.e-12) && (ic <= 10)) 
	e1    = (shoot - am1 - eccentricity*sin(shoot)) / ...
			(1.0 - eccentricity*cos(shoot));
    shoot = shoot - e1;
    ic    = ic + 1;
end

if (ic >= 10)
    disp ('warning ** subroutine kepler did not converge in 10 iterations');
end

%eccentric = shoot;
E = shoot;
%%%%%%%%%%%%%%%%%%%%%%%%%%%%%%%%%%%%%%%%%%%%%%
sE   = sin(E);
cE   = cos(E);
c3   = sqrt(EARTH_GRAVITY/a)/(1. - exc*cE);

%     state vector

statvec = [[a*(cE - exc), a*c1*sE, 0]*orb2iner', [-c3*sE, c1*c3*cE, 0]*orb2iner'];

== matlab function untitled1/Subsystem1/Convert Terrestrial Geocentric to Speherical coordinates ECEF2LLA ==
  data: geoc input; spherical output
function spherical  = rectangular_to_spherical (geoc)
% [spherical] = rectangular_to_spherical (geoc)
%	Function to transform rectangular terrestrial
%	geocentric coordinates in spherical coordinates
%	(longitude, geocentric latitude and distance).
%
% Inputs:
%   geoc
%   		geocentric rectangular coordinates vector in meters
%           (1) geocentric position x (m)
%           (2) geocentric position y (m)
%           (3) geocentric position z (m)
%
% Outputs:
%	spherical
%		Geocentric coordinates vector:
%			1 = east longitude (rad)
%			2 = geocentric latitude (rad)
%			3 = geocentric distance (meters)
%
% Authors:
%   Valdemir Carrara            May/09        Matlab

px = geoc(1);
py = geoc(2);
pz = geoc(3);
ws = px*px + py*py;
rw = sqrt(ws + pz *pz);
lg = atan2(py, px);
lt = atan2(pz, sqrt(ws));
spherical = [lg, lt, rw];

== matlab function untitled1/Subsystem1/ECI to ECEF  ==
  data: tesig input; xterrestrial output; xi input
function xterrestrial  = inertial_to_terrestrial (tesig, xi)
% [xterrestrial] = inertial_to_terrestrial (tesig, xi)
%	The function inertial_to_terrestrial transforms geocentric
%	inertial state vector into geocentric
%	terrestrial coordinates (referred to
%	Greenwich).
%
% Input:
%	tesig
%		Greenwich sidereal time in radians.
%	xi
%		geocentric inertial position vector.
%       (1) inertial geocentric position x (m)
%       (2) inertial geocentric position y (m)
%       (3) inertial geocentric position z (m)
%       (4) inertial geocentric velocity x (m/s)
%       (5) inertial geocentric velocity y (m/s)
%       (6) inertial geocentric velocity z (m/s)
%
% Output:
%	xterrestrial
%		corresponding geocentric terrestrial vector.
%
% Authors:
%	Helio/Valder/Valdemir-aug. 1981 - version 1.0
%	Helio		-july 1989 - version 1.1
%	Valdemir Carrara		july 2005		(C version)
%   Valdemir Carrara            March/09        Matlab
coan    =  cos(tesig);
sian    =  sin(tesig);
rot_mat =  [ coan, sian, 0 ;
            -sian, coan, 0 ; 
                0,    0, 1];

xterrestrial_ = [xi(1:3); xi(4:6)]*rot_mat';
xterrestrial  = [xterrestrial_(1,:) xterrestrial_(2,:)];

== matlab function untitled1/MATLAB Function ==
  data: initial_condition input; dfdt output; f_vec input
function dfdt  = eq_propagate(initial_condition, f_vec)
% u=3.9865*10^14;
u=3.9865*10^14;
% Re=6378.14;         % Earth Radius
Re = 6378137; % earth radius in m

dfdt = zeros(size(initial_condition));

%x=x
%x1=dx/dt
%dx1/dt = d^2(x)/dt
% f_vec = [rand(1)*0 rand(1)*0 rand(1)*0]';

x1 = initial_condition(4); % x1 = dx/dt
y1 = initial_condition(5); % y1 = dy/dt
z1 = initial_condition(6); % z1 = dz/dt
x  = initial_condition(1); % x
y  = initial_condition(2); % y
z  = initial_condition(3); % z

m  = initial_condition(7); % mass

r=sqrt(x^2+y^2+z^2);

% % %   Keplar Motion Equatnion
% % %  => r_dd + u/(r^3)r_ = 0 => r_dd = -u/(r^3)r_
dfdt(1) = x1;
dfdt(2) = y1;
dfdt(3) = z1;
dfdt(4) = -u*x/r^3 + f_vec(1,1);
dfdt(5) = -u*y/r^3 + f_vec(2,1);
dfdt(6) = -u*z/r^3 + f_vec(3,1);
dfdt(7) = 0;
end

== matlab function untitled1/MATLAB Function2 ==
  data: kep input; state output
% function [X, Y, Z, Vx, Vy, Vz] = Kepler2Carts(alt, ecc, inc, w, nu, RAAN)
function state = Kepler2Carts(kep)
%--------------------------------------------------------------------------------------------------------%
%
% 			USAGE: Conversion of Keplerian Classic Orbital Elements into geocentric-equatorial reference system OXYZ
%
% 			AUTHOR: Thameur Chebbi(PhD)		E-MAIL: chebbythamer@gmail.com
%
% 			DATE: 01,Oct,2020
%
% 			DESCIPTION:      This function is created to convert the classical 
%               		     orbital elements to cartesian position and velocity 
%		       		         parameters of any satellite orbit in the geocentric-equatorial
%                            reference system.
%
% 			INPUT:
%           kep0 =>
% 			alt:    Altitude.....................(Km)							
% 			ecc:    Eccentricity											    
% 			inc:	Inclination..................(rad)							
% 			w:	    Argument of perigee..........(rad)	
% 			nu:	    Satellite position...........(rad)							
% 			RAAN:	Right Asc. of Ascending Node.(rad)							
%
% 			OUTPUT:
%			Position Components: 		
% 			[X  Y  Z ]....(Km)
%
%			Velocity Components:
% 			[Vx Vy Vz]....(Km/s) 														
%
alt  = kep(1,1);    ecc  = kep(1,2);
inc  = kep(1,3);    w    = kep(1,4);
nu   = kep(1,5);    RAAN = kep(1,6);
%%---------------------------- Constants ----------------------------------------------%
% mu_earth = 3.986 * 10^5; % Earth Gravitational Constant
mu_earth = 3.9865 * 10^14; % Earth Gravitational Constant
% re = 6378.1; % earth radius in km
re = 6378137; % earth radius in m
%
%%--------------------------------------------------------------------------------------
a = alt + re;
p = a*(1-ecc ^2);
r_0 = p / (1 + ecc * cos(nu));
%
%%--------------- Coordinates in the perifocal reference system Oxyz -----------------%
%
% position vector coordinates
x = r_0 * cos(nu);
y = r_0 * sin(nu);
%
%
% velocity vector coordinates
Vx_ = -(mu_earth/p)^(1/2) * sin(nu);
Vy_ = (mu_earth/p)^(1/2) * (ecc + cos(nu));
%
%
%%-------------- the geocentric-equatorial reference system OXYZ ---------------------%
%
% position vector components X, Y, and Z
X = (cos(RAAN) * cos(w) - sin(RAAN) * sin(w) * cos(inc)) * x + (-cos(RAAN) * sin(w) - sin(RAAN) * cos(w) * cos(inc)) * y;
Y = (sin(RAAN) * cos(w) + cos(RAAN) * sin(w) * cos(inc)) * x + (-sin(RAAN) * sin(w) + cos(RAAN) * cos(w) * cos(inc)) * y;
Z = (sin(w) * sin(inc)) * x + (cos(w) * sin(inc)) * y;
% velocity vector components X', Y', and Z'
Vx = (cos(RAAN) * cos(w) - sin(RAAN) * sin(w) * cos(inc)) * Vx_ + (-cos(RAAN) * sin(w) - sin(RAAN) * cos(w) * cos(inc)) * Vy_;
Vy = (sin(RAAN) * cos(w) + cos(RAAN) * sin(w) * cos(inc)) * Vx_ + (-sin(RAAN) * sin(w) + cos(RAAN) * cos(w) * cos(inc)) * Vy_;
Vz = (sin(w) * sin(inc)) * Vx_ + (cos(w) * sin(inc)) * Vy_;

state = [X,Y,Z,Vx,Vy,Vz,10];

end

== matlab function untitled1/MATLAB Function4 ==
  settings: updateMethod=DISCRETE
  data: vec input; y output; kep_flg output; t input; tran_flg output
function [y, kep_flg, tran_flg] = fcn(vec, t)
ft = 10000;
dt = 1000;


persistent first_flg
persistent tran_flg_save


if isempty(first_flg)
    tran_flg_save = 0;
    first_flg = 1;
end

if tran_flg_save == 0
    if( t <= ft )
        y = 0*vec;
    else
        tran_flg_save = tran_flg_save + 1;
        y = 0*vec;
    end
    kep_flg  = 1;

elseif tran_flg_save == 1
    if ((t>ft) && (t<=(ft+dt)))%firing
        y = 1*vec;
        kep_flg  = 0;
    else
        y = 0*vec;
        kep_flg  = 1;
        tran_flg_save = tran_flg_save + 1;
    end

elseif tran_flg_save == 2
    y = 0*vec;
    kep_flg  = 1;
else
    y = 0*vec;
    kep_flg  = 1;
end

tran_flg = tran_flg_save;

% if ((t>=ft) && (t<=(ft+dt)))
%     y = 1*vec;
%     kep_flg  = 0;
%     tran_flg = 1;
% else
%     y = 0*vec;
%     kep_flg  = 1;
%     tran_flg_save = 0;
% end

end

== matlab function untitled1/MATLAB Function5 ==
  settings: updateMethod=DISCRETE
  data: statv input; kepel output; kep_flg input
function kepel  = statvec_kepel (statv, kep_flg)
%	The function statvec_kepel transforms the state vector statv
%	into the corresponding keplerian elements in the
%	same reference system.
%
% Input:
%	statv
%		state vector in meters and meters/second.
%
% Output:
%	statvec_kepel
%		vector containing the keplerian elements:
%		(1) - semimajor axis of the orbit in meters.
%		(2) - eccentricity.
%		(3) - inclination in radians.
%		(4) - right ascension of ascending node in radians.
%		(5) - argument of perigee in radians.
%		(6) - mean anomaly in radians.
persistent kepel_save
persistent first_flg

if isempty(first_flg)
    kepel_save = [0 0 0 0 0 0];
    first_flg = 1;
end

EARTH_GRAVITY	= 3.9860064e+14;		% Earth's gravitational constant (m**3/s**2)

if kep_flg == 1
    xp     = [statv(1),statv(2),statv(3)];
    xv     = [statv(4),statv(5),statv(6)];
    r      = sqrt(xp*xp');
    vq     = xv*xv';
    ainv   = 2.0/(r) - vq/EARTH_GRAVITY;

    h      = cross(xp, xv);
    hm     = sqrt(h*h');
    if (hm < 1.e-10)
        disp (' *** Message from function statvec_kepel: *** ');
        disp (' There are no keplerian elements corresponding to this state vector');
        kepel = [0, 0, 0, 0, 0, 0];
    else
        h      = h/hm;
        incl   = acos(h(3));
        raan   = atan2(h(1), -h(2));
        d      = xp*xv' / EARTH_GRAVITY;
        esene  = d * sqrt(EARTH_GRAVITY*ainv);
        ecose  = 1 - r*ainv;
        exc    = sqrt(esene*esene + ecose*ecose);
        E      = atan2(esene, ecose);
        mean   = mod (E - esene, 2*pi);
        an = [0 0 0];
        if mean < 0
            mean = mean + 2*pi;
        end
        if exc < 1.e-10
            arpe = 0;
        else
            dp     = 1./r - ainv;
            ev     = dp*xp - d*xv;
            abev   = sqrt(ev*ev');
            ev     = ev/abev;
            an(1)  = cos(raan);
            an(2)  = sin(raan);
            an(3)  = 0;
            fi     = ev*cross(h, an)';
            arpe = acos(ev*an');
            if fi < 0
                arpe  =  -arpe + 2*pi;
            end
        end

        kepel = [(1./ainv), exc, incl, raan, arpe, mean];
        kepel_save = kepel;
%         T = 2*pi*sqrt((a*a*a)/(EARTH_GRAVITY));
    end
else

    kepel = kepel_save;
    T = 0;
end


end

== matlab function untitled1/Greenwich Aparent Mean Sideral Time ==
  data: diju input; gwst output; time input
function gwst  = gst (diju, time)
% [gwst] = gst (diju, time)
%   The function gst furnishes the greenwich aparent mean 
%   sidereal time referred to the J2000.0 equator and equinox.
% inputs:
%   diju
%       Modified Julian Date in days, referred to 1950.0.
%   time
%       UT1 time complement in seconds.
% outputs:
%   gwst
%       Greenwich aparent sidereal time in radians
%
% Valdemir Carrara, Apr, 2003
%

tsj = (diju-18262.5)/36525;
tsgo = (24110.54841 + (8640184.812866 + 9.3104e-2*tsj - 6.2e-6*tsj*tsj)*tsj)*pi/43200;
tetp = 7.292116e-5;		% velocidade angular da Terra (rd/s) mean angular velocity of the Earth
gwst = mod(tsgo + time*tetp, 2*pi);
% reference site
% https://www2.mps.mpg.de/homes/fraenz/systems/systems2art/node10.html
%      if (gwst<0) gwst = gwst + 2*pi

== matlab function untitled1/Ephemerides Date1/Modified Julian Date (mjd) ==
  data: dmy input; diju output
function diju  =  djm (dmy)
% [diju] = djm (day, month, year)
%    The function djm furnishes the Modified Julian
%    Date with reference to the day, month and year,
%    at zero hours of the day.
% inputs:
%   dmy(1): day, day of the month
%   dmy(2): month, month of the year
%   dmy(3): year

% outputs:
%   diju
%       Modified Julian Date in days, referred to 1950.0. 
%
% Valdemir Carrara, Apr, 2003
%

diju = 367*dmy(3) + dmy(1) - 712269 + fix(275*dmy(2)/9)- fix(7*(dmy(3)+fix((dmy(2)+9)/12))/4);

== matlab function untitled1/MATLAB Function9 ==
  data: ECEF2ECI input; ECI_vecX output; ECI_vecY output; ECI_vecZ output; ECEF_vecX output; ECEF_vecY output; ECEF_vecZ output; LVLH_vecX output; LVLH_vecY output; LVLH_vecZ output; ECI2LVLH input; ECI2BODY input; BODY_vecX output; BODY_vecY output; BODY_vecZ output
function [ ECI_vecX,  ECI_vecY,  ECI_vecZ,...
          ECEF_vecX, ECEF_vecY, ECEF_vecZ,...
          LVLH_vecX, LVLH_vecY, LVLH_vecZ,...
          BODY_vecX, BODY_vecY, BODY_vecZ] = ...
          fcn(ECEF2ECI, ECI2LVLH, ECI2BODY)

ECI_vecX  = [5000000, 0, 0]';
ECI_vecY  = [0, 5000000, 0]';
ECI_vecZ  = [0, 0, 5000000]';

ECEF_vecX = ECEF2ECI'*ECI_vecX;
ECEF_vecY = ECEF2ECI'*ECI_vecY;
ECEF_vecZ = ECEF2ECI'*ECI_vecZ;

sc=0.5;
LVLH_vecX = ECI2LVLH'*ECI_vecX*sc;
LVLH_vecY = ECI2LVLH'*ECI_vecY*sc;
LVLH_vecZ = ECI2LVLH'*ECI_vecZ*sc;

BODY_vecX = ECI2BODY'*ECI_vecX*sc;
BODY_vecY = ECI2BODY'*ECI_vecY*sc;
BODY_vecZ = ECI2BODY'*ECI_vecZ*sc;
% BODY_vecX = LVLH2BODY(:,1)*500000;
% BODY_vecY = LVLH2BODY(:,2)*500000;
% BODY_vecZ = LVLH2BODY(:,3)*500000;


end

== matlab function untitled1/Ephemerides Date1/Modified Julian Date (mjd0) ==
  data: dmy input; diju output
function diju  =  djm (dmy)
% [diju] = djm (day, month, year)
%    The function djm furnishes the Modified Julian
%    Date with reference to the day, month and year,
%    at zero hours of the day.
% inputs:
%   dmy(1): day, day of the month
%   dmy(2): month, month of the year
%   dmy(3): year

% outputs:
%   diju
%       Modified Julian Date in days, referred to 1950.0. 
%
% Valdemir Carrara, Apr, 2003
%

diju = 367*dmy(3) + dmy(1) - 712269 + fix(275*dmy(2)/9)- fix(7*(dmy(3)+fix((dmy(2)+9)/12))/4);

== matlab function untitled1/Ephemerides Date1/Modified Julian Date (mjd1) ==
  data: dmy input; diju output
function diju  =  djm (dmy)
% [diju] = djm (day, month, year)
%    The function djm furnishes the Modified Julian
%    Date with reference to the day, month and year,
%    at zero hours of the day.
% inputs:
%   dmy(1): day, day of the month
%   dmy(2): month, month of the year
%   dmy(3): year

% outputs:
%   diju
%       Modified Julian Date in days, referred to 1950.0. 
%
% Valdemir Carrara, Apr, 2003
%

diju = 367*dmy(3) + dmy(1) - 712269 + fix(275*dmy(2)/9)- fix(7*(dmy(3)+fix((dmy(2)+9)/12))/4);
